simulink model "power_netsim2"  (Simulink 6.0)
settings: Solver=ode23s  SolverMode=SingleTasking  StartTime=0.0  StopTime=0.06  RelTol=1e-3  AbsTol=1e-6
libraries: powerlib x8, powerlib_extras x1
settings Model: Creator=patrice  LastModifiedBy=batserve  ExtModeTrigMode=oneshot  ExtModeArmWhenConnect=off  ExtModeAutoUpdateStatusClock=off
settings DataIOCC: LimitDataPoints=off  SignalLoggingName=sigsOut
settings OptimizationCC: BooleanDataType=off
settings DebuggingCC: SolverPrmCheckMsg=none
settings HardwareCC: TargetUnknown=on
settings RTWCC: TemplateMakefile=grt_unix.tmf

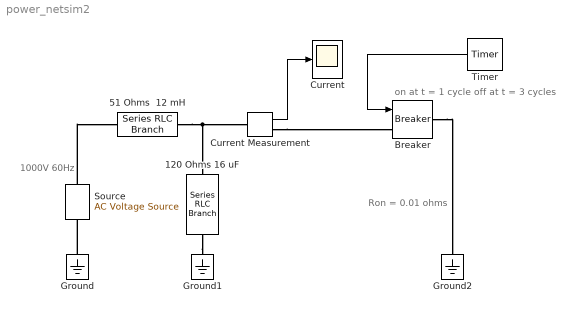
== system power_netsim2 ==
  note: Ron = 0.01 ohms
  note: on at t = 1 cycle
      | off at t = 3 cycles
  note: 1000V
      |  60Hz
  "120 Ohms 16 uF " : powerlib/Elements/Series RLC Branch  Orientation=down  PhysicalDomain=powersysdomain  SubClassName=unknown  PortType=p1  LConnTagsString=__new0  RConnTagsString=__new0  Resistance=120  Inductance=0  Capacitance=16e-06  Measurements=None
  51 Ohms  12 mH : powerlib/Elements/Series RLC Branch  PhysicalDomain=powersysdomain  SubClassName=unknown  PortType=p1  LConnTagsString=__new0  RConnTagsString=__new0  Resistance=51  Inductance=12e-03  Capacitance=inf  Measurements=None
  "Breaker " : powerlib/Elements/Breaker  BreakerResistance=0.01  InitialState=0  SnubberResistance=inf  SnubberCapacitance=0  SwitchingTimes="[ 4/60  5/60 ]"  External=on  Measurements=None
      settings: AttributesFormatString=\n
  Current : Scope
      settings: TickLabels=on  TimeRange=0.06  YMin=-20  YMax=20  DataFormat=Array
  Current Measurement : powerlib/Measurements/Current Measurement  Tag=PoWeRsYsTeMmEaSuReMeNt  PhasorSimulation=off  OutputType=Magnitude  PSBequivalent=0
  Ground : powerlib/Elements/Ground  Orientation=down  PhysicalDomain=powersysdomain  SubClassName=unknown  PortType=p1  LConnTagsString=a
  Ground1 : powerlib/Elements/Ground  Orientation=down  PhysicalDomain=powersysdomain  SubClassName=unknown  PortType=p1  LConnTagsString=a
  Ground2 : powerlib/Elements/Ground  Orientation=down  PhysicalDomain=powersysdomain  SubClassName=unknown  PortType=p1  LConnTagsString=a
  Source : powerlib/Electrical Sources/AC Voltage Source  Description=source block  Orientation=up  Amplitude=1000  Phase=0  Frequency=60  SampleTime=0  Measurements=None
      settings: AttributesFormatString=\n
  Timer : powerlib_extras/Control  Blocks/Timer  Orientation=left  t=[0 1/60 3/60]  e=[0 1 0 ]
  wires:
  Current Measurement/1 -> Current/1
  Timer/1 -> "Breaker "/1
  connections:
  51 Ohms  12 mH/RConn1 -- Current Measurement/LConn1 -- "120 Ohms 16 uF "/LConn1
  "120 Ohms 16 uF "/RConn1 -- Ground1/LConn1
  "Breaker "/RConn1 -- Ground2/LConn1
  Current Measurement/RConn1 -- "Breaker "/LConn1
  Source/RConn1 -- 51 Ohms  12 mH/LConn1
  Ground/LConn1 -- Source/LConn1
